simulink model "gps_rascunho"  (R2024b)
settings: Solver=VariableStepAuto  StartTime=0.0  StopTime=tsim  RelTol=1e-3
values from neighbouring files (symbols this model uses):
  gg0 = 0    [Grupo3RP1.m]    (also in all_values.m; init.m; main.m; new_A_B_lambda.m)
  sample_time_gps = 1/freq_amos_gps    (= 0.2)    [main.m]
  u0 = u0*0.51444    (= 27.985536)    [Grupo3RP1.m]    (also in all_values.m; init.m = [da0, dr0]; untitled2.m)
undefined symbols (not defined in the file or in its folder): E0, N0, Vwind
libraries: simulink x4
settings Model: Creator=quico  LastModifiedBy=ruben

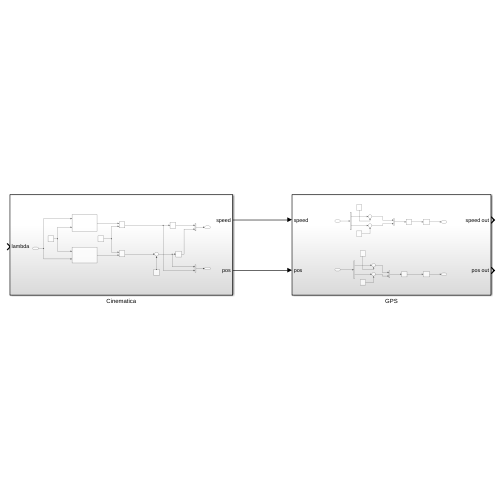
[thumbnail: Simulink's stored preview of the top-level diagram]
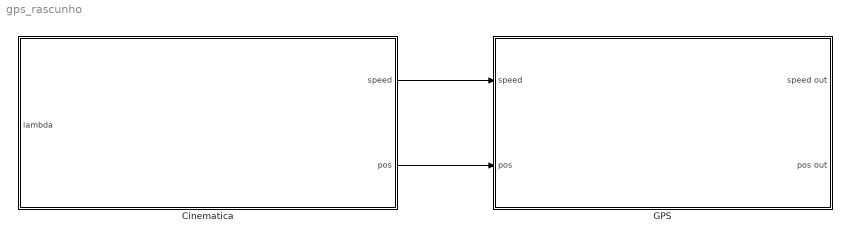
== system gps_rascunho ==
  Cinematica : Subsystem
  GPS : Subsystem
  wires:
  Cinematica/1(speed) -> GPS/1(speed)
  Cinematica/2(pos) -> GPS/2(pos)

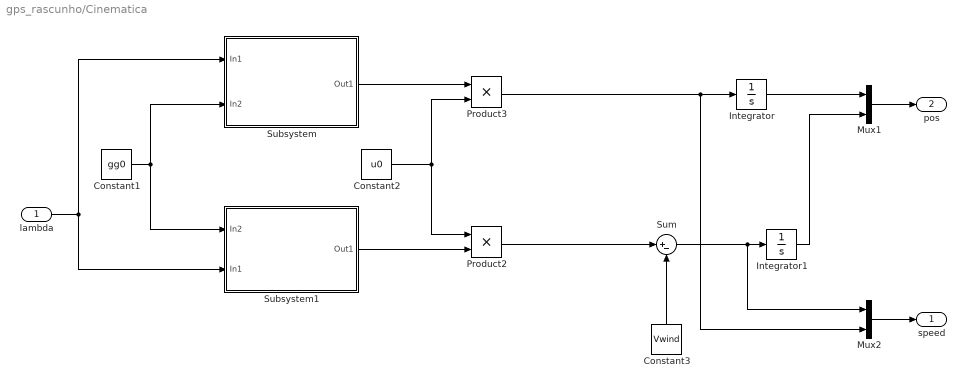
== system gps_rascunho/Cinematica ==
  lambda : Inport
  Constant1 : Constant  Value=gg0
  Constant2 : Constant  Value=u0
  Constant3 : Constant  Value=Vwind
  Integrator : Integrator  InitialCondition=E0
  Integrator1 : Integrator  InitialCondition=N0
  Mux1 : Mux  Inputs=2
  Mux2 : Mux  Inputs=2
  Product2 : Product
  Product3 : Product
  Subsystem : Subsystem
  Subsystem1 : Subsystem
  Sum : Sum  Inputs=|+-
  speed : Outport
  pos : Outport  Port=2
  wires:
  lambda/1 -> Subsystem1/2(In1), Subsystem/1(In1)
  Constant2/1 -> Product3/2, Product2/1
  Product3/1 -> Mux2/2, Integrator/1
  Product2/1 -> Sum/1
  Constant3/1 -> Sum/2
  Sum/1 -> Mux2/1, Integrator1/1
  Integrator/1 -> Mux1/1
  Integrator1/1 -> Mux1/2
  Mux2/1 -> speed/1
  Mux1/1 -> pos/1
  Subsystem/1(Out1) -> Product3/1
  Constant1/1 -> Subsystem/2(In2), Subsystem1/1(In2)
  Subsystem1/1(Out1) -> Product2/2

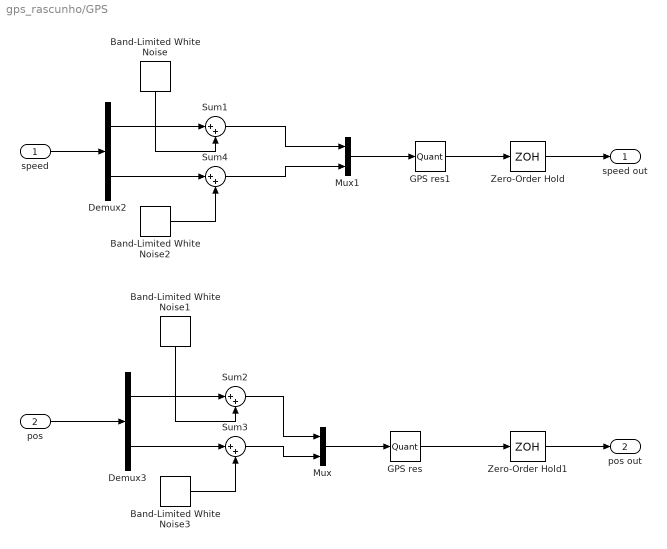
== system gps_rascunho/GPS ==
  speed : Inport
  pos : Inport  Port=2
  Band-Limited White Noise : simulink/Sources/Band-Limited White Noise  Cov=sample_time_gps*0.1*0.1  Ts=sample_time_gps  seed=[18414]
  Band-Limited White Noise1 : simulink/Sources/Band-Limited White Noise  Cov=sample_time_gps*2.5*2.5  Ts=sample_time_gps  seed=[678549302]
  Band-Limited White Noise2 : simulink/Sources/Band-Limited White Noise  Cov=sample_time_gps*0.1*0.1  Ts=sample_time_gps  seed=[7634853920]
  Band-Limited White Noise3 : simulink/Sources/Band-Limited White Noise  Cov=sample_time_gps*2.5*2.5  Ts=sample_time_gps  seed=[678954302]
  Demux2 : Demux  Outputs=2
  Demux3 : Demux  Outputs=2
  GPS res : Quantizer
  GPS res1 : Quantizer  QuantizationInterval=0.01
  Mux : Mux  Inputs=2
  Mux1 : Mux  Inputs=2
  Sum{1..4} (4 alike) : Sum  Inputs=|++
  Zero-Order Hold : ZeroOrderHold  SampleTime=sample_time_gps
  Zero-Order Hold1 : ZeroOrderHold  SampleTime=sample_time_gps
  speed out : Outport
  pos out : Outport  Port=2
  wires:
  Mux/1 -> GPS res/1
  GPS res/1 -> Zero-Order Hold1/1
  GPS res1/1 -> Zero-Order Hold/1
  Mux1/1 -> GPS res1/1
  speed/1 -> Demux2/1
  Demux2/1 -> Sum1/1
  Demux2/2 -> Sum4/1
  Band-Limited White Noise/1 -> Sum1/2
  Band-Limited White Noise2/1 -> Sum4/2
  Demux3/2 -> Sum3/1
  pos/1 -> Demux3/1
  Band-Limited White Noise3/1 -> Sum3/2
  Demux3/1 -> Sum2/1
  Band-Limited White Noise1/1 -> Sum2/2
  Sum2/1 -> Mux/1
  Sum3/1 -> Mux/2
  Sum4/1 -> Mux1/2
  Sum1/1 -> Mux1/1
  Zero-Order Hold/1 -> speed out/1
  Zero-Order Hold1/1 -> pos out/1

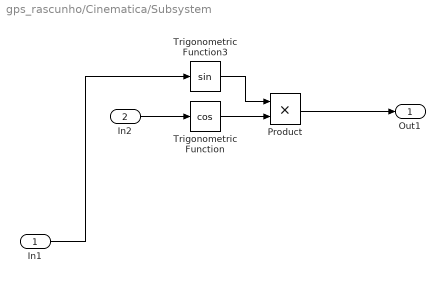
== system gps_rascunho/Cinematica/Subsystem ==
  In1 : Inport
  In2 : Inport  Port=2
  Product : Product
  Trigonometric Function : Trigonometry  Operator=cos
  Trigonometric Function3 : Trigonometry
  Out1 : Outport
  wires:
  Trigonometric Function3/1 -> Product/1
  Trigonometric Function/1 -> Product/2
  In1/1 -> Trigonometric Function3/1
  Product/1 -> Out1/1
  In2/1 -> Trigonometric Function/1

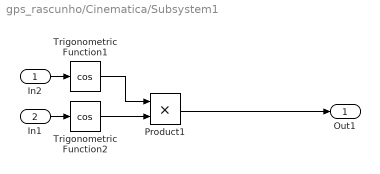
== system gps_rascunho/Cinematica/Subsystem1 ==
  In2 : Inport
  In1 : Inport  Port=2
  Product1 : Product
  Trigonometric Function1 : Trigonometry  Operator=cos
  Trigonometric Function2 : Trigonometry  Operator=cos
  Out1 : Outport
  wires:
  Trigonometric Function2/1 -> Product1/2
  Trigonometric Function1/1 -> Product1/1
  In2/1 -> Trigonometric Function1/1
  In1/1 -> Trigonometric Function2/1
  Product1/1 -> Out1/1
